simulink model "computeTau"  (Simulink 7.7)
settings: Solver=FixedStepDiscrete  StartTime=0.0  StopTime=5  FixedStep=0.01  RelTol=1e-3
PreLoadFcn:
  | robotName = 'icubGazeboSim';
  | localName = 'SimulinkiCubGazeboSim';
InitFcn:
  | robotName = 'icubGazeboSim';
  | localName = 'SimulinkiCubGazeboSim';
libraries: WBCLibrary x10, utility x1, simulink x1, dspsigops x1
settings Model: Creator=iron  LastModifiedBy=iron

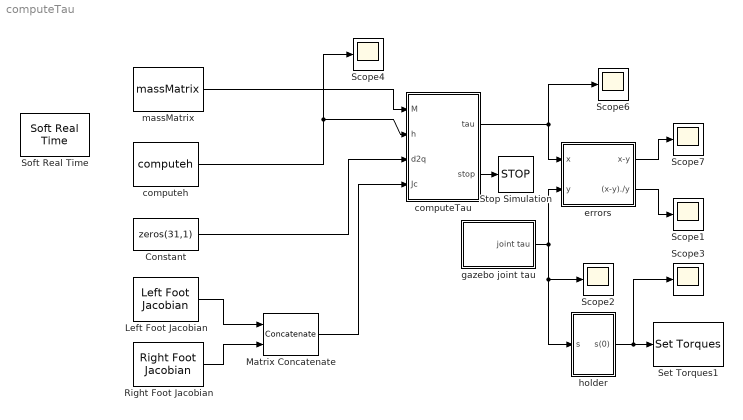
== system computeTau ==
  Constant : Constant  Value=zeros(31,1)
  Left Foot Jacobian : WBCLibrary/wholeBodyModel/Jacobians/Left Foot Jacobian  SystemSampleTime=-1  robotName=robotName  localName=localName
  Matrix Concatenate : Concatenate  Mode=Multidimensional array
  Right Foot Jacobian : WBCLibrary/wholeBodyModel/Jacobians/Right Foot Jacobian  SystemSampleTime=-1  robotName=robotName  localName=localName
  Scope{1..4,6..7} (6 alike) : Scope
      Scope1 settings: YMin=-60  YMax=60
      Scope2 settings: YMin=-5.5  YMax=3  SaveName=ScopeData2
      Scope3 settings: YMin=-5.5  YMax=3  SaveName=ScopeData3
      Scope4 settings: YMax=2  SaveName=ScopeData4
      Scope6 settings: YMin=-60  YMax=60  SaveName=ScopeData6
      Scope7 settings: YMin=-60  YMax=60  SaveName=ScopeData7
  Set Torques1 : WBCLibrary/wholeBodyActuators/Set Torques  SystemSampleTime=-1  val=6  robotName=robotName  localName=localName
  Soft Real Time : utility/Soft Real Time  x=1
  Stop Simulation : Stop
  computeTau : Stateflow chart  TreatAsAtomicUnit=on
  computeh : WBCLibrary/wholeBodyModel/Dynamics/computeh  SystemSampleTime=-1  val=7  robotname=robotName  localname=localName
  errors : Subsystem
  gazebo joint tau : Subsystem
  holder : Subsystem
  massMatrix : WBCLibrary/wholeBodyModel/Dynamics/massMatrix  SystemSampleTime=-1  val=8  robotname=robotName  localname=localName
  wires:
  massMatrix/1 -> computeTau/1(M)
  computeh/1 -> computeTau/2(h), Scope4/1
  Left Foot Jacobian/1 -> Matrix Concatenate/1
  Right Foot Jacobian/1 -> Matrix Concatenate/2
  Matrix Concatenate/1 -> computeTau/4(Jc)
  gazebo joint tau/1(joint tau) -> Scope2/1, holder/1(s), errors/2(y)
  holder/1(s(0)) -> Scope3/1, Set Torques1/1
  computeTau/2(stop) -> Stop Simulation/1
  computeTau/1(tau) -> Scope6/1, errors/1(x)
  Constant/1 -> computeTau/3(d2q)
  errors/2((x-y)./y) -> Scope1/1
  errors/1(x-y) -> Scope7/1

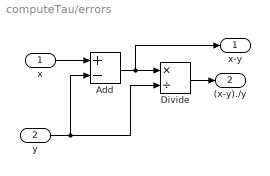
== system computeTau/errors ==
  x : Inport
  y : Inport  Port=2
  Add : Sum  Inputs=+-
  Divide : Product  Inputs=*/
  x-y : Outport
  (x-y)./y : Outport  Port=2
  wires:
  Add/1 -> Divide/1, x-y/1
  x/1 -> Add/1
  y/1 -> Add/2, Divide/2
  Divide/1 -> (x-y)./y/1

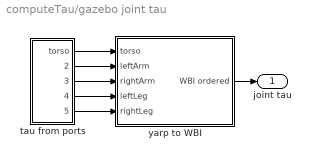
== system computeTau/gazebo joint tau ==
  tau from ports : Subsystem
  yarp to WBI : Subsystem
  joint tau : Outport
  wires:
  tau from ports/2(leftArm) -> yarp to WBI/2(leftArm)
  tau from ports/1(torso) -> yarp to WBI/1(torso)
  tau from ports/5(rightLeg) -> yarp to WBI/5(rightLeg)
  tau from ports/3(rightArm) -> yarp to WBI/3(rightArm)
  tau from ports/4(leftLeg) -> yarp to WBI/4(leftLeg)
  yarp to WBI/1(WBI ordered) -> joint tau/1

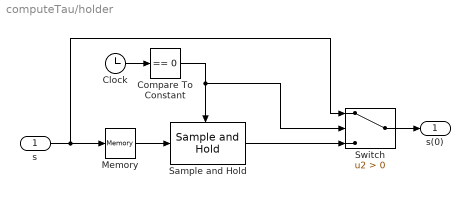
== system computeTau/holder ==
  s : Inport
  Clock : Clock
      settings: Decimation=10
  Compare To Constant : simulink/Logic and Bit Operations/Compare To Constant  SystemSampleTime=-1  relop===  const=0  LogicOutDataTypeMode=boolean
  Memory : Memory
  Sample and Hold : dspsigops/Sample and Hold  SystemSampleTime=-1  trig=Falling edge  initCond=0  latchinput=off
  Switch : Switch  Criteria=u2 > Threshold
  s(0) : Outport
  wires:
  s/1 -> Switch/1, Memory/1
  Clock/1 -> Compare To Constant/1
  Compare To Constant/1 -> Sample and Hold/Trigger, Switch/2
  Sample and Hold/1 -> Switch/3
  Switch/1 -> s(0)/1
  Memory/1 -> Sample and Hold/1

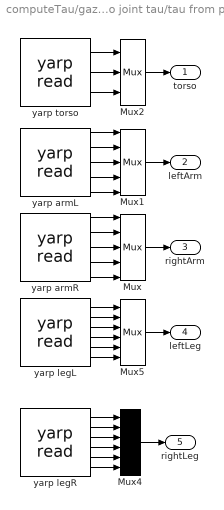
== system computeTau/gazebo joint tau/tau from ports ==
  Mux : Mux  Inputs=5
  Mux1 : Mux  Inputs=5
  Mux2 : Mux  Inputs=3
  Mux4 : Mux  Inputs=6
  Mux5 : Mux  Inputs=6
  yarp armL : WBCLibrary/Utilities/yarp read  from='/icubGazeboSim/left_arm/analog:o/torques'  to='/tmp2:i'  num=5
  yarp armR : WBCLibrary/Utilities/yarp read  from='/icubGazeboSim/right_arm/analog:o/torques'  to='/tmp3:i'  num=5
  yarp legL : WBCLibrary/Utilities/yarp read  from='/icubGazeboSim/left_leg/analog:o/torques'  to='/tmp4:i'  num=6
  yarp legR : WBCLibrary/Utilities/yarp read  from='/icubGazeboSim/right_leg/analog:o/torques'  to='/tmp5:i'  num=6
  yarp torso : WBCLibrary/Utilities/yarp read  from='/icubGazeboSim/torso/analog:o/torques'  to='/tmp1:i'  num=3
  torso : Outport
  leftArm : Outport  Port=2
  rightArm : Outport  Port=3
  leftLeg : Outport  Port=4
  rightLeg : Outport  Port=5
  wires:
  yarp armR/1 -> Mux/1
  yarp armR/2 -> Mux/2
  yarp armR/3 -> Mux/3
  yarp armR/4 -> Mux/4
  yarp armR/5 -> Mux/5
  yarp armL/1 -> Mux1/1
  yarp armL/2 -> Mux1/2
  yarp armL/3 -> Mux1/3
  yarp armL/4 -> Mux1/4
  yarp armL/5 -> Mux1/5
  yarp torso/1 -> Mux2/1
  yarp torso/2 -> Mux2/2
  yarp torso/3 -> Mux2/3
  yarp legL/1 -> Mux5/1
  yarp legL/2 -> Mux5/2
  yarp legL/3 -> Mux5/3
  yarp legL/4 -> Mux5/4
  yarp legL/5 -> Mux5/5
  yarp legL/6 -> Mux5/6
  yarp legR/1 -> Mux4/1
  yarp legR/2 -> Mux4/2
  yarp legR/3 -> Mux4/3
  yarp legR/4 -> Mux4/4
  yarp legR/5 -> Mux4/5
  yarp legR/6 -> Mux4/6
  Mux2/1 -> torso/1
  Mux1/1 -> leftArm/1
  Mux/1 -> rightArm/1
  Mux5/1 -> leftLeg/1
  Mux4/1 -> rightLeg/1

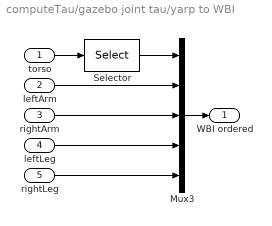
== system computeTau/gazebo joint tau/yarp to WBI ==
  torso : Inport
  leftArm : Inport  Port=2
  rightArm : Inport  Port=3
  leftLeg : Inport  Port=4
  rightLeg : Inport  Port=5
  Mux3 : Mux  Inputs=5
  Selector : Selector  InputPortWidth=3  IndexOptions=Index vector (dialog)  Indices=[3 2 1]  OutputSizes=1
  WBI ordered : Outport
  wires:
  Selector/1 -> Mux3/1
  torso/1 -> Selector/1
  leftArm/1 -> Mux3/2
  rightArm/1 -> Mux3/3
  Mux3/1 -> WBI ordered/1
  leftLeg/1 -> Mux3/4
  rightLeg/1 -> Mux3/5

== matlab function computeTau ==
  data: M input double; h input double; d2q input double; tau output double; Jc input double; stop output double
function [tau, stop] = fcn(M, h, d2q, Jc)

% Francesco Nori
% Genova 6 Marzo 2014
% CODYCO project
%
% This code computes the torques tau necessary to obtain a desired
% acceleration d2q in a kinematic chain with contacts. These 
% computations are described in (DelPrete,2013) Ph.D. thesis
% and can be found also in [Aghili 2005; Righetti et al. 2011]. It can
% be shown that:
%
% tau = pinv(Nc' S') Nc (M d2q  + h)  
%
% with Nc = (I-pinv(Jc)Jc) and the constraints being described as:
%
% Jc dq = 0
%
% Jc d2q + dJcdq= 0

[~, n] = size(Jc);
n = n - 6;
S = [zeros(n,6) eye(n)];

Nc = (eye(n+6)-pinv(Jc, 1e-2)*Jc);
tau = pinv(Nc' * S', 1e-2) * Nc *(M * d2q  + h);

stop = norm(tau)>50;
